simulink model "CA_DPIC_model"  (R2022b)
settings: Solver=ode45  StartTime=0.0  StopTime=10  RelTol=1e-3  AbsTol=1e-6
values from neighbouring files (symbols this model uses):
  linA = [      zeros(3, 3), eye(3, 3);      - m * l, zeros(3, 3) ... (first row only)    [MainForProject.m]
  linB = [zeros(3, 1); m * [1; 0; 0]]    [MainForProject.m]
  linC = [0, 1, zeros(1, 4)]    [MainForProject.m]
  linD = 0    [MainForProject.m]
  Q0 = zeros(6, 1)    [MainForProject.m]
settings Model: PacingRate=0.001000  Creator=utente  LastModifiedBy=utente
settings DataIOCC: ExternalInput=[functA functB]  InitialState=Q0

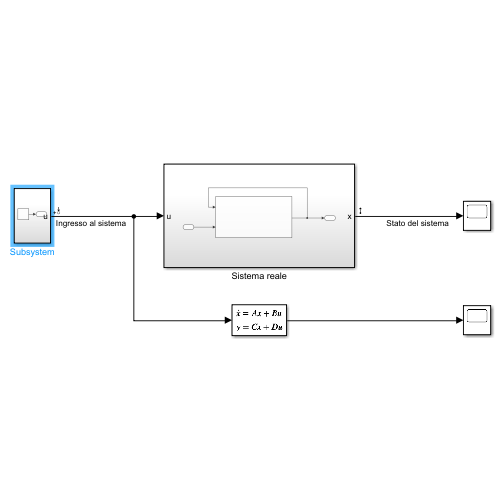
[thumbnail: Simulink's stored preview of the top-level diagram]
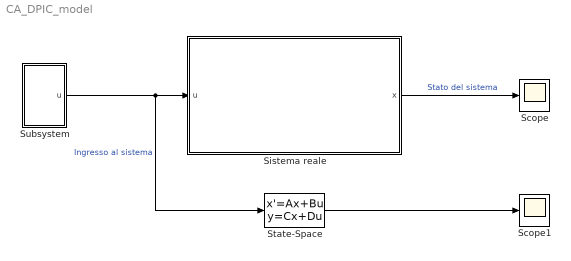
== system CA_DPIC_model ==
  Scope : Scope
  Scope1 : Scope
  Sistema reale : Subsystem
  State-Space : StateSpace  A=linA  B=linB  C=linC  D=linD  InitialCondition=Q0
  Subsystem : Subsystem
  wires:
  Sistema reale/1(x) -> Scope/1  "Stato del sistema"
  Subsystem/1(u) -> State-Space/1, Sistema reale/1(u)  "Ingresso al sistema"
  State-Space/1 -> Scope1/1

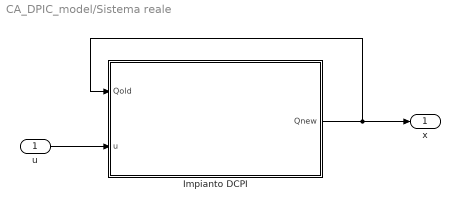
== system CA_DPIC_model/Sistema reale ==
  u : Inport
  Impianto DCPI : Subsystem
  x : Outport
  wires:
  u/1 -> Impianto DCPI/2(u)
  Impianto DCPI/1(Qnew) -> x/1, Impianto DCPI/1(Qold)

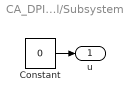
== system CA_DPIC_model/Subsystem ==
  Constant : Constant  Value=0
  u : Outport
  wires:
  Constant/1 -> u/1

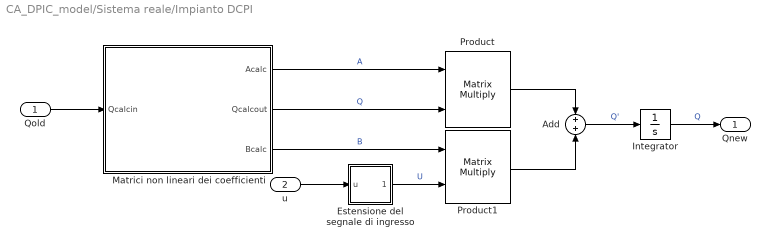
== system CA_DPIC_model/Sistema reale/Impianto DCPI ==
  Qold : Inport
  u : Inport  Port=2
  Add : Sum
  Estensione del segnale di ingresso : Subsystem
  Integrator : Integrator  InitialCondition=Q0
  Matrici non lineari dei coefficienti : Subsystem
  Product : Product  Multiplication=Matrix(*)
  Product1 : Product  Multiplication=Matrix(*)
  Qnew : Outport
  wires:
  Matrici non lineari dei coefficienti/2(Qcalcout) -> Product/2  "Q"
  Matrici non lineari dei coefficienti/1(Acalc) -> Product/1  "A"
  Estensione del segnale di ingresso/1(Ucalc) -> Product1/2  "U"
  Add/1 -> Integrator/1  "Q'"
  Matrici non lineari dei coefficienti/3(Bcalc) -> Product1/1  "B"
  u/1 -> Estensione del segnale di ingresso/1(u)
  Integrator/1 -> Qnew/1  "Q"
  Qold/1 -> Matrici non lineari dei coefficienti/1(Qcalcin)
  Product/1 -> Add/1
  Product1/1 -> Add/2

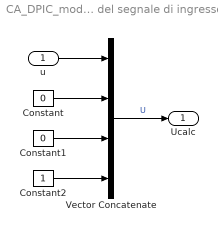
== system CA_DPIC_model/Sistema reale/Impianto DCPI/Estensione del segnale di ingresso ==
  u : Inport
  Constant : Constant  Value=0
  Constant1 : Constant  Value=0
  Constant2 : Constant
  Vector Concatenate : Concatenate  NumInputs=4
  Ucalc : Outport
  wires:
  Constant1/1 -> Vector Concatenate/3
  Constant2/1 -> Vector Concatenate/4
  Constant/1 -> Vector Concatenate/2
  Vector Concatenate/1 -> Ucalc/1  "U"
  u/1 -> Vector Concatenate/1

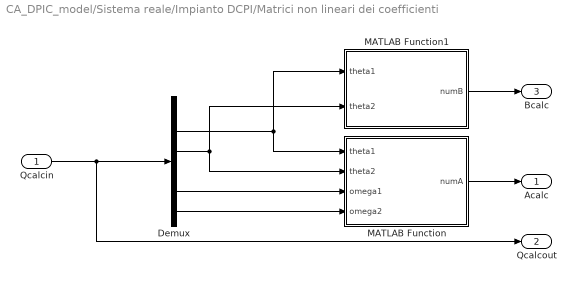
== system CA_DPIC_model/Sistema reale/Impianto DCPI/Matrici non lineari dei coefficienti ==
  Qcalcin : Inport
  Demux : Demux  Outputs=6
  MATLAB Function : MATLAB Function  TreatAsAtomicUnit=on
  MATLAB Function1 : MATLAB Function  TreatAsAtomicUnit=on
  Acalc : Outport
  Qcalcout : Outport  Port=2
  Bcalc : Outport  Port=3
  wires:
  MATLAB Function/1(numA) -> Acalc/1
  MATLAB Function1/1(numB) -> Bcalc/1
  Qcalcin/1 -> Demux/1, Qcalcout/1
  Demux/6 -> MATLAB Function/4(omega2)
  Demux/5 -> MATLAB Function/3(omega1)
  Demux/3 -> MATLAB Function1/2(theta2), MATLAB Function/2(theta2)
  Demux/2 -> MATLAB Function1/1(theta1), MATLAB Function/1(theta1)

== matlab function CA_DPIC_model/Sistema reale/Impianto DCPI/Matrici non lineari dei coefficienti/MATLAB Function1 ==
  data: theta1 input double; numB output double size=[6 4]; theta2 input double
function numB = calculateB(theta1, theta2)
    numB = functB(theta1, theta2);
end

== matlab function CA_DPIC_model/Sistema reale/Impianto DCPI/Matrici non lineari dei coefficienti/MATLAB Function ==
  data: theta1 input; numA output double size=[6 6]; theta2 input; omega1 input double; omega2 input double
function numA = calculateA(theta1, theta2, omega1, omega2)
    numA = functA(theta1, theta2, omega1, omega2);
end
